simulink model "SF049A_LoaMgr"  (R2013b)
settings: Solver=FixedStepDiscrete  SolverMode=SingleTasking  StartTime=0.0  StopTime=1  FixedStep=0.002  RelTol=1e-3
values from neighbouring files (symbols this model uses):
  CURRMEASLOAMTGTNMASK_CNT_U08 = DataDict.Constant    [SF049A_LoaMgr_DataDict.m]
  IVTRLOAMTGTNMASK_CNT_U08 = DataDict.Constant    [SF049A_LoaMgr_DataDict.m]
  LOAMAXSLEW_ULSPERSEC_F32 = DataDict.Constant    [SF049A_LoaMgr_DataDict.m]
  LoaMgrCurrIvtrMtgtnRate = DataDict.Calibration    [SF049A_LoaMgr_DataDict.m]
  LoaMgrCurrIvtrMtgtnSca = DataDict.Calibration    [SF049A_LoaMgr_DataDict.m]
  LoaMgrCurrIvtrMtgtnScaZeroEna = DataDict.Calibration    [SF049A_LoaMgr_DataDict.m]
  LoaMgrCurrMeasIdptSig0Resp = DataDict.Calibration    [SF049A_LoaMgr_DataDict.m]
  LoaMgrCurrMeasIdptSig1Resp = DataDict.Calibration    [SF049A_LoaMgr_DataDict.m]
  LoaMgrCurrMeasIdptSig2Resp = DataDict.Calibration    [SF049A_LoaMgr_DataDict.m]
  LoaMgrCurrMeasIdptSigFltThd = DataDict.Calibration    [SF049A_LoaMgr_DataDict.m]
  LoaMgrCurrMeasMtgtnRate = DataDict.Calibration    [SF049A_LoaMgr_DataDict.m]
  LoaMgrCurrMeasMtgtnSca = DataDict.Calibration    [SF049A_LoaMgr_DataDict.m]
  LoaMgrCurrMeasMtgtnScaZeroEna = DataDict.Calibration    [SF049A_LoaMgr_DataDict.m]
  LoaMgrFadeOutStRate = DataDict.Calibration    [SF049A_LoaMgr_DataDict.m]
  LoaMgrHwTqIdptSig0NoTqLoaResp = DataDict.Calibration    [SF049A_LoaMgr_DataDict.m]
  LoaMgrHwTqIdptSig1NoTqLoaResp = DataDict.Calibration    [SF049A_LoaMgr_DataDict.m]
  LoaMgrHwTqIdptSig2Resp = DataDict.Calibration    [SF049A_LoaMgr_DataDict.m]
  LoaMgrHwTqIdptSig4Resp = DataDict.Calibration    [SF049A_LoaMgr_DataDict.m]
  LoaMgrHwTqIdptSigFltThd = DataDict.Calibration    [SF049A_LoaMgr_DataDict.m]
  LoaMgrHwTqLoaAvlResp = DataDict.Calibration    [SF049A_LoaMgr_DataDict.m]
  LoaMgrIvtrIdptSig0Resp = DataDict.Calibration    [SF049A_LoaMgr_DataDict.m]
  LoaMgrIvtrIdptSig1Resp = DataDict.Calibration    [SF049A_LoaMgr_DataDict.m]
  LoaMgrIvtrIdptSig2Resp = DataDict.Calibration    [SF049A_LoaMgr_DataDict.m]
  LoaMgrIvtrIdptSigFltThd = DataDict.Calibration    [SF049A_LoaMgr_DataDict.m]
  LoaMgrIvtrMtgtnRate = DataDict.Calibration    [SF049A_LoaMgr_DataDict.m]
  LoaMgrIvtrMtgtnSca = DataDict.Calibration    [SF049A_LoaMgr_DataDict.m]
  LoaMgrIvtrMtgtnScaZeroEna = DataDict.Calibration    [SF049A_LoaMgr_DataDict.m]
  LoaMgrLimdStRate = DataDict.Calibration    [SF049A_LoaMgr_DataDict.m]
  LoaMgrLimdStSca = DataDict.Calibration    [SF049A_LoaMgr_DataDict.m]
  LoaMgrMotAgAvlSnsrlsResp = DataDict.Calibration    [SF049A_LoaMgr_DataDict.m]
  LoaMgrMotAgIdptSig0NoSnsrlsResp = DataDict.Calibration    [SF049A_LoaMgr_DataDict.m]
  LoaMgrMotAgIdptSig1NoSnsrlsResp = DataDict.Calibration    [SF049A_LoaMgr_DataDict.m]
  LoaMgrMotAgIdptSig2Resp = DataDict.Calibration    [SF049A_LoaMgr_DataDict.m]
  LoaMgrMotAgIdptSig3Resp = DataDict.Calibration    [SF049A_LoaMgr_DataDict.m]
  LoaMgrMotAgIdptSigFltThd = DataDict.Calibration    [SF049A_LoaMgr_DataDict.m]
  LoaMgrMotAgMtgtnRate = DataDict.Calibration    [SF049A_LoaMgr_DataDict.m]
  LoaMgrMotAgMtgtnSca = DataDict.Calibration    [SF049A_LoaMgr_DataDict.m]
  LoaMgrMotAgMtgtnScaZeroEna = DataDict.Calibration    [SF049A_LoaMgr_DataDict.m]
  LOASCAONE_ULS_F32 = DataDict.Constant    [SF049A_LoaMgr_DataDict.m]
  LOASCAZERO_ULS_F32 = DataDict.Constant    [SF049A_LoaMgr_DataDict.m]
  LOASTIMDTSHTDWN_CNT_U08 = DataDict.Constant    [SF049A_LoaMgr_DataDict.m]
  LOASTNORM_CNT_U08 = DataDict.Constant    [SF049A_LoaMgr_DataDict.m]
  LOASTSWMTGTN_CNT_U08 = DataDict.Constant    [SF049A_LoaMgr_DataDict.m]
  MAXCURRMEASIDPTSIGALLWD_CNT_U08 = DataDict.Constant    [SF049A_LoaMgr_DataDict.m]
  MAXHWTQIDPTSIGALLWD_CNT_U08 = DataDict.Constant    [SF049A_LoaMgr_DataDict.m]
  MAXIVTRIDPTSIGALLWD_CNT_U08 = DataDict.Constant    [SF049A_LoaMgr_DataDict.m]
  MAXMOTAGMECLIDPTSIGALLWD_CNT_U08 = DataDict.Constant    [SF049A_LoaMgr_DataDict.m]
  NODEBSTEP_CNT_U16 = DataDict.Constant    [SF049A_LoaMgr_DataDict.m]
undefined symbols (not defined in the file or in its folder): LoaSt1, NtcNr1, NtcSts1, SigQlfr1
libraries: simulink x43, NxtrMin x4, NxtrMax x4, NxtrLim x2
(part 1 of 8)
settings Model: Creator=TZ5743  LastModifiedBy=dzvc93
settings SolverCC: AutoInsertRateTranBlk=on  InsertRTBMode=Always
settings DataIOCC: LimitDataPoints=off  SaveFormat=Structure  ReturnWorkspaceOutputs=on
settings OptimizationCC: BlockReduction=off  InlineParams=on  ZeroExternalMemoryAtStartup=off  ZeroInternalMemoryAtStartup=off  OptimizeModelRefInitCode=on  LifeSpan=1
settings DebuggingCC: SignalInfNanChecking=error  SignalRangeChecking=warning  UnderspecifiedInitializationDetection=Simplified  SolverPrmCheckMsg=error  InheritedTsInSrcMsg=error  DiscreteInheritContinuousMsg=error  SingleTaskRateTransMsg=error  TasksWithSamePriorityMsg=error  SigSpecEnsureSampleTimeMsg=error  CheckMatrixSingularityMsg=error  ParameterUnderflowMsg=error  ParameterPrecisionLossMsg=error  ParameterTunabilityLossMsg=error  FixptConstUnderflowMsg=warning  FixptConstOverflowMsg=warning  VectorMatrixConversionMsg=error  SignalLabelMismatchMsg=error  UnconnectedInputMsg=error  UnconnectedOutputMsg=error  UnconnectedLineMsg=error  SFcnCompatibilityMsg=error  UniqueDataStoreMsg=warning  BusObjectLabelMismatch=error  RootOutportRequireBusObject=error  AssertControl=DisableAll  ModelReferenceIOMsg=error  ModelReferenceVersionMismatchMessage=warning  ModelReferenceIOMismatchMessage=error  ModelReferenceCSMismatchMessage=warning  ModelReferenceDataLoggingMessage=error  StateNameClashWarn=warning  StrictBusMsg=ErrorOnBusTreatedAsVector  NonBusSignalsTreatedAsBus=error  SFUnexpectedBacktrackingDiag=error  SFInvalidInputDataAccessInChartInitDiag=error  SFNoUnconditionalDefaultTransitionDiag=error  SFTransitionOutsideNaturalParentDiag=error  SFUnconditionalTransitionShadowingDiag=error  SFUndirectedBroadcastEventsDiag=error
settings ModelReferenceCC: ModelReferenceNumInstancesAllowed=Single
settings RTWCC: SystemTargetFile=autosar.tlc  GenCodeOnly=on  TemplateMakefile=ert_default_tmf  Description=AUTOSAR  GenerateReport=on  ProcessScript=autosar_make_rtw_hook  LaunchReport=on
settings CodeAppCC: GenerateComments=off  IgnoreCustomStorageClasses=off  CustomSymbolStrType=$N$R$M  CustomSymbolStrBlkIO=$N$M  SimulinkBlockComments=off
settings STFCustomTargetCC: ParMdlRefBuildCompliant=on  CompOptLevelCompliant=on  IncludeMdlTerminateFcn=off  CombineOutputUpdateFcns=on  SuppressErrorStatus=on  ERTFirstTimeCompliant=on  ERTCustomFileBanners=on  SupportNonFinite=off  SupportComplex=off  SupportContinuousTime=off  SupportNonInlinedSFcns=off  MATLABClassNameForMDSCustomization=Simulink.SoftwareTarget.ERTCustomization  AutosarCompliant=on  GRTInterface=off  SystemTargetFile=autosar.tlc
settings ERTTargetCC: CodeReplacementLibrary=ANSI_C  ConcurrentExecutionCompliant=off  IncludeMdlTerminateFcn=off  SuppressErrorStatus=on  SupportNonFinite=off  SupportComplex=off  ModelStepFunctionPrototypeControlCompliant=off  CPPClassGenCompliant=off  AutosarCompliant=on  InlinedParameterPlacement=NonHierarchical  ERTCustomFileTemplate=example_file_process.tlc  EnableUserReplacementTypes=on

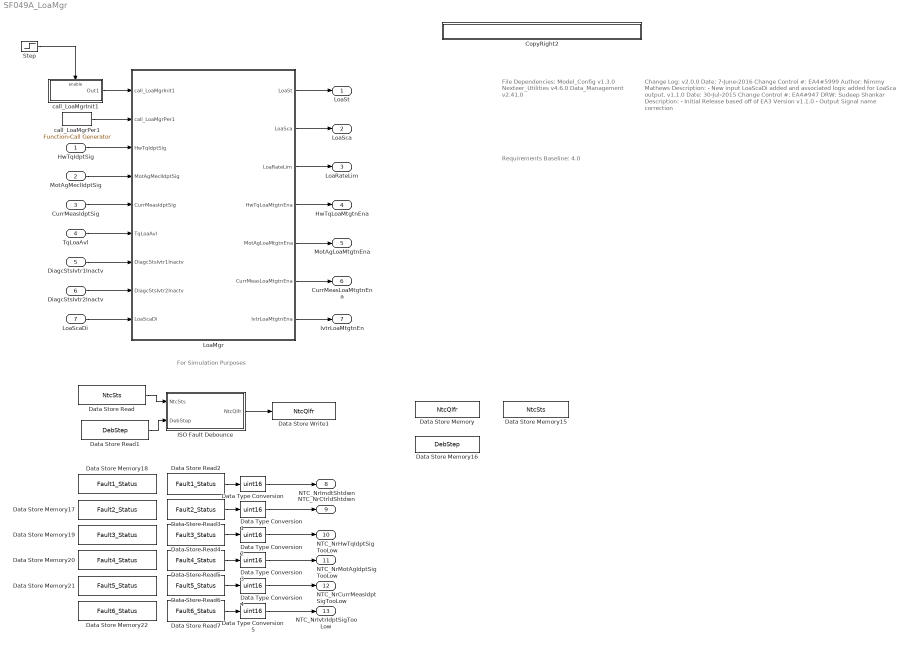
== system SF049A_LoaMgr ==
  note: File Dependencies:
      |
      | Model_Config v1.3.0
      | Nexteer_Utilities v4.6.0
      | Data_Management v2.41.0
  note: Requirements Baseline: 4.0
  note: Change Log:
      | v2.0.0
      | Date: 7-June-2016
      | Change Control #: 	EA4#5999
      | Author:  Nimmy Mathews
      | Description:
      | - New input LoaScaDi added and associated logic added for
      | LoaSca output.
      |
      | v1.1.0
      | Date: 30-Jul-2015
      | Change Control #: EA4#947
      | DRW:  Sudeep Shankar
      | Description:
      | - Initial Release based off of EA3 Version v1.1.0
      | - Output Signal name correction
  note: For Simulation Purposes
  HwTqIdptSig : Inport  RequirementInfo="{'linktype_rmi_doors' '0000bab3 (/E-STEER Core/SubSystem Specifications/Application Functions/SF049A Loss of Assist Manager)' '#SF049A_12' 'true' 'REQ:  SF049A_12' '' } %GIDa_c0ada7cc_2a84_41fc_944b_6b17ef65ea9c"
  MotAgMeclIdptSig : Inport  RequirementInfo="{'linktype_rmi_doors' '0000bab3 (/E-STEER Core/SubSystem Specifications/Application Functions/SF049A Loss of Assist Manager)' '#SF049A_14' 'true' 'REQ:  SF049A_14' '' } %GIDa_73372f4d_c568_47db_aad1_8b4638be1747"  Port=2
  CurrMeasIdptSig : Inport  RequirementInfo="{'linktype_rmi_doors' '0000bab3 (/E-STEER Core/SubSystem Specifications/Application Functions/SF049A Loss of Assist Manager)' '#SF049A_43' 'true' 'REQ:  SF049A_43' '' } %GIDa_84af9224_d287_43ff_b284_7e5ed6dfb324"  Port=3
  TqLoaAvl : Inport  RequirementInfo="{'linktype_rmi_doors' '0000bab3 (/E-STEER Core/SubSystem Specifications/Application Functions/SF049A Loss of Assist Manager)' '#SF049A_13' 'true' 'REQ:  SF049A_13' '' } %GIDa_93076217_93fd_4cef_a21d_6480a5a63a27"  Port=4
  DiagcStsIvtr1Inactv : Inport  RequirementInfo="{'linktype_rmi_doors' '0000bab3 (/E-STEER Core/SubSystem Specifications/Application Functions/SF049A Loss of Assist Manager)' '#SF049A_44' 'true' 'REQ:  SF049A_44' '' } %GIDa_3739eb85_24f0_476e_b882_4900d0ef3f73"  Port=5
  DiagcStsIvtr2Inactv : Inport  RequirementInfo="{'linktype_rmi_doors' '0000bab3 (/E-STEER Core/SubSystem Specifications/Application Functions/SF049A Loss of Assist Manager)' '#SF049A_184' 'true' 'REQ:  SF049A_184' '' } %GIDa_5f578b66_4982_413b_90dc_34bab3afd1d1"  Port=6
  LoaScaDi : Inport  RequirementInfo="{'linktype_rmi_doors' '0000bab3 (/E-STEER Core/SubSystem Specifications/Application Functions/SF049A Loss of Assist Manager)' '#SF049A_202' 'true' 'REQ:  SF049A_202' '' } %GIDa_13ee9f09_c993_4f8a_825d_b1ce3d1d2719"  Port=7
  CopyRight2 : Subsystem  Description=|  mask(Copyright Information){none=on}
      | Copyright info block.                                               
      |                                                                     
      | Place copyright information at the top of every subsystem in design.
      mask prompts: none "No parameters"
      mask help: Place copyright information at the top of every subsystem in design.
      mask Display:
      | NxtrConf = 'Nexteer Confidential';
      | 
      | sys = bdroot; %handle for the current model ("system")
      | first = get_param(sys,'Created');
      | if(isempty(first))
      |     first = datestr(now,'yyyy');
      | else
      |     first = first(end-3:end);  %year is last four digits
      | end
      | 
      | last = get_param(sys,'LastModifiedDate');
      | if isempty(last)
      |     last = datestr(now,'yyyy');
      | else
      |     last = last(end-3:end);
      | end
      | 
      | if strcmp(first,last)
      |     fprintf('%s -- Copyright %s Nexteer',NxtrConf,first)
      | else
      |     fprintf('%s -- %s%s- %s Nexteer',NxtrConf,char(169),first,last)
      | end
  Data Store Memory : DataStoreMemory  DataStoreName=NtcQlfr  OutDataTypeStr=uint8
  Data Store Memory15 : DataStoreMemory  DataStoreName=NtcSts  InitialValue=NtcSts1.NTCSTS_PREPASSD
  Data Store Memory16 : DataStoreMemory  DataStoreName=DebStep
  Data Store Memory17 : DataStoreMemory  DataStoreName=Fault2_Status  InitialValue=NtcSts1.NTCSTS_PASSD  OutDataTypeStr=Enum: NtcSts1
  Data Store Memory18 : DataStoreMemory  DataStoreName=Fault1_Status  InitialValue=NtcSts1.NTCSTS_PASSD  OutDataTypeStr=Enum: NtcSts1
  Data Store Memory19 : DataStoreMemory  DataStoreName=Fault3_Status  InitialValue=NtcSts1.NTCSTS_PASSD  OutDataTypeStr=Enum: NtcSts1
  Data Store Memory20 : DataStoreMemory  DataStoreName=Fault4_Status  InitialValue=NtcSts1.NTCSTS_PASSD  OutDataTypeStr=Enum: NtcSts1
  Data Store Memory21 : DataStoreMemory  DataStoreName=Fault5_Status  InitialValue=NtcSts1.NTCSTS_PASSD  OutDataTypeStr=Enum: NtcSts1
  Data Store Memory22 : DataStoreMemory  DataStoreName=Fault6_Status  InitialValue=NtcSts1.NTCSTS_PASSD  OutDataTypeStr=Enum: NtcSts1
  Data Store Read : DataStoreRead  DataStoreName=NtcSts  SampleTime=0.004
  Data Store Read1 : DataStoreRead  DataStoreName=DebStep  SampleTime=0.004
  Data Store Read2 : DataStoreRead  DataStoreName=Fault1_Status  SampleTime=.004
  Data Store Read3 : DataStoreRead  DataStoreName=Fault2_Status  SampleTime=.004
  Data Store Read4 : DataStoreRead  DataStoreName=Fault3_Status  SampleTime=.004
  Data Store Read5 : DataStoreRead  DataStoreName=Fault4_Status  SampleTime=.004
  Data Store Read6 : DataStoreRead  DataStoreName=Fault5_Status  SampleTime=.004
  Data Store Read7 : DataStoreRead  DataStoreName=Fault6_Status  SampleTime=0.004
  Data Store Write1 : DataStoreWrite  DataStoreName=NtcQlfr
  Data Type Conversion{,1..5} (6 alike) : DataTypeConversion  OutDataTypeStr=uint16
  ISO Fault Debounce : Subsystem
  LoaMgr : Subsystem
  Step : Step  Time=.001  Before=1  After=0  SampleTime=0
  call_LoaMgrInit1 : Subsystem  TreatAsAtomicUnit=on
  call_LoaMgrPer1 : simulink/Ports & Subsystems/Function-Call Generator  RequirementInfo="{'linktype_rmi_doors' '0000bab3 (/E-STEER Core/SubSystem Specifications/Application Functions/SF049A Loss of Assist Manager)' '#SF049A_28' 'true' 'REQ:  SF049A_28' '' } %GIDa_b45244a2_9238_4316_a679_a7195a05364e"  sample_time=0.004  numberOfIterations=1
  LoaSt : Outport  RequirementInfo="{'linktype_rmi_doors' '0000bab3 (/E-STEER Core/SubSystem Specifications/Application Functions/SF049A Loss of Assist Manager)' '#SF049A_16' 'true' 'REQ:  SF049A_16' '' } %GIDa_93bae52a_8cb1_4bd9_a2c4_d588b7d059cf"
  LoaSca : Outport  RequirementInfo="{'linktype_rmi_doors' '0000bab3 (/E-STEER Core/SubSystem Specifications/Application Functions/SF049A Loss of Assist Manager)' '#SF049A_17' 'true' 'REQ:  SF049A_17' '' } %GIDa_8c460775_12f6_4528_9f51_57ca189e85fc"  Port=2
  LoaRateLim : Outport  RequirementInfo="{'linktype_rmi_doors' '0000bab3 (/E-STEER Core/SubSystem Specifications/Application Functions/SF049A Loss of Assist Manager)' '#SF049A_18' 'true' 'REQ:  SF049A_18' '' } %GIDa_ffab9872_1ea4_4ffd_9e16_324c719cb008"  Port=3
  HwTqLoaMtgtnEna : Outport  RequirementInfo="{'linktype_rmi_doors' '0000bab3 (/E-STEER Core/SubSystem Specifications/Application Functions/SF049A Loss of Assist Manager)' '#SF049A_46' 'true' 'REQ:  SF049A_46' '' } %GIDa_b272817b_3ff3_4259_b745_ea4cd35b806a"  Port=4
  MotAgLoaMtgtnEna : Outport  RequirementInfo="{'linktype_rmi_doors' '0000bab3 (/E-STEER Core/SubSystem Specifications/Application Functions/SF049A Loss of Assist Manager)' '#SF049A_47' 'true' 'REQ:  SF049A_47' '' } %GIDa_98224876_72c1_4d11_a238_725dcb00f091"  Port=5
  CurrMeasLoaMtgtnEna : Outport  RequirementInfo="{'linktype_rmi_doors' '0000bab3 (/E-STEER Core/SubSystem Specifications/Application Functions/SF049A Loss of Assist Manager)' '#SF049A_48' 'true' 'REQ:  SF049A_48' '' } %GIDa_771c3727_c0e3_4c42_9260_a180eb374e5c"  Port=6
  IvtrLoaMtgtnEn : Outport  RequirementInfo="{'linktype_rmi_doors' '0000bab3 (/E-STEER Core/SubSystem Specifications/Application Functions/SF049A Loss of Assist Manager)' '#SF049A_49' 'true' 'REQ:  SF049A_49' '' } %GIDa_ccb9de9c_ade8_4e48_bfad_57a91e3cbf19"  Port=7
  NTC_NrImdtShtdwn : Outport  Port=8
  NTC_NrCtrldShtdwn : Outport  Port=9
  NTC_NrHwTqIdptSigTooLow : Outport  Port=10
  NTC_NrMotAgIdptSigTooLow : Outport  Port=11
  NTC_NrCurrMeasIdptSigTooLow : Outport  Port=12
  NTC_NrIvtrIdptSigTooLow : Outport  Port=13
  wires:
  HwTqIdptSig/1 -> LoaMgr/3(HwTqIdptSig)
  MotAgMeclIdptSig/1 -> LoaMgr/4(MotAgMeclIdptSig)
  CurrMeasIdptSig/1 -> LoaMgr/5(CurrMeasIdptSig)
  DiagcStsIvtr1Inactv/1 -> LoaMgr/7(DiagcStsIvtr1Inactv)
  TqLoaAvl/1 -> LoaMgr/6(TqLoaAvl)
  DiagcStsIvtr2Inactv/1 -> LoaMgr/8(DiagcStsIvtr2Inactv)
  LoaMgr/7(IvtrLoaMtgtnEna) -> IvtrLoaMtgtnEn/1
  LoaMgr/6(CurrMeasLoaMtgtnEna) -> CurrMeasLoaMtgtnEna/1
  LoaMgr/5(MotAgLoaMtgtnEna) -> MotAgLoaMtgtnEna/1
  LoaMgr/4(HwTqLoaMtgtnEna) -> HwTqLoaMtgtnEna/1
  LoaMgr/3(LoaRateLim) -> LoaRateLim/1
  LoaMgr/2(LoaSca) -> LoaSca/1
  LoaMgr/1(LoaSt) -> LoaSt/1
  call_LoaMgrPer1/1 -> LoaMgr/2(call_LoaMgrPer1)
  call_LoaMgrInit1/1(Out1) -> LoaMgr/1(call_LoaMgrInit1)
  Step/1 -> call_LoaMgrInit1/Enable
  Data Store Read2/1 -> Data Type Conversion/1
  Data Type Conversion/1 -> NTC_NrImdtShtdwn/1
  Data Store Read3/1 -> Data Type Conversion1/1
  Data Type Conversion1/1 -> NTC_NrCtrldShtdwn/1
  Data Store Read4/1 -> Data Type Conversion2/1
  Data Type Conversion2/1 -> NTC_NrHwTqIdptSigTooLow/1
  Data Type Conversion3/1 -> NTC_NrMotAgIdptSigTooLow/1
  Data Type Conversion4/1 -> NTC_NrCurrMeasIdptSigTooLow/1
  Data Store Read5/1 -> Data Type Conversion3/1
  Data Store Read6/1 -> Data Type Conversion4/1
  Data Type Conversion5/1 -> NTC_NrIvtrIdptSigTooLow/1
  Data Store Read7/1 -> Data Type Conversion5/1
  ISO Fault Debounce/1(NtcQlfr) -> Data Store Write1/1
  Data Store Read/1 -> ISO Fault Debounce/1(NtcSts)
  Data Store Read1/1 -> ISO Fault Debounce/2(DebStep)
  LoaScaDi/1 -> LoaMgr/9(LoaScaDi)

== system SF049A_LoaMgr/CopyRight2 ==

== system SF049A_LoaMgr/ISO Fault Debounce ==
  note: Note:
      |
      | - "ISO Fault Debounce Design" Simulink block intent to use here for Simulation purpose only. Do not Code this block
  NtcSts : Inport
  DebStep : Inport  Port=2
  Constant : Constant  Value=false
  CopyRight2 : Subsystem  Description=|  mask(Copyright Information){none=on}
      | Copyright info block.                                               
      |                                                                     
      | Place copyright information at the top of every subsystem in design.
      mask prompts: none "No parameters"
      mask help: Place copyright information at the top of every subsystem in design.
      mask Display:
      | NxtrConf = 'Nexteer Confidential';
      | 
      | sys = bdroot; %handle for the current model ("system")
      | first = get_param(sys,'Created');
      | first = first(end-3:end);  %year is last four digits
      | 
      | last = get_param(sys,'LastModifiedDate');
      | if isempty(last)
      |     last = datestr(now,'yyyy');
      | else
      |     last = last(end-3:end);
      | end
      | 
      | if strcmp(first,last)
      |     fprintf('%s -- Copyright %s Nexteer',NxtrConf,first)
      | else
      |     fprintf('%s -- %s%s- %s Nexteer',NxtrConf,char(169),first,last)
      | end
  Data Type Conversion : DataTypeConversion
  DiagMgr : Subsystem  RequirementInfo="{'linktype_rmi_doors' '00007fee (/E-STEER Core/SubSystem Specifications/Application Functions/SF004B Assist Summation and Limiting- Current)' '#SF004B_271' 'true' 'REQ:  SF004B_271' '' ; 'linktype_rmi_doors' '00007fee (/E-STEER Core/SubSystem Specifications/Application Functions/SF004B Assist Summation and Limiting- Current)' '#SF004B_270' 'true' 'REQ:  SF004B_270' '' ; 'linktype_rmi_doors' '00007fee (/E-STEER Core/SubSystem Specifications/Application Functions/SF004B Assist Summation and Limiting- Current)' '#SF004B_272' 'true' 'REQ:  SF004B_272' '' ; 'linktype_rmi_doors' '00007fee (/E-STEER Core/SubSystem Specifications/Application Functions/SF004B Assist Summation and Limiting- Current)' '#SF004B_273' 'true' 'REQ:  SF004B_273' '' } %GIDa_8ac3e521_cc41_436f_a252_177cc8f755d2"
  Ground : Ground
  Scope2 : Scope
      settings: SaveName=ScopeData2
  Terminator : Terminator
  NtcQlfr : Outport
  wires:
  Ground/1 -> DiagMgr/3(SvcClr)
  DebStep/1 -> DiagMgr/2(DebStep), Scope2/1
  NtcSts/1 -> DiagMgr/1(NtcSts)
  Constant/1 -> DiagMgr/4(Recoverable)
  Data Type Conversion/1 -> NtcQlfr/1
  DiagMgr/1(Qualifier) -> Data Type Conversion/1
  DiagMgr/2(ErrAcc) -> Terminator/1

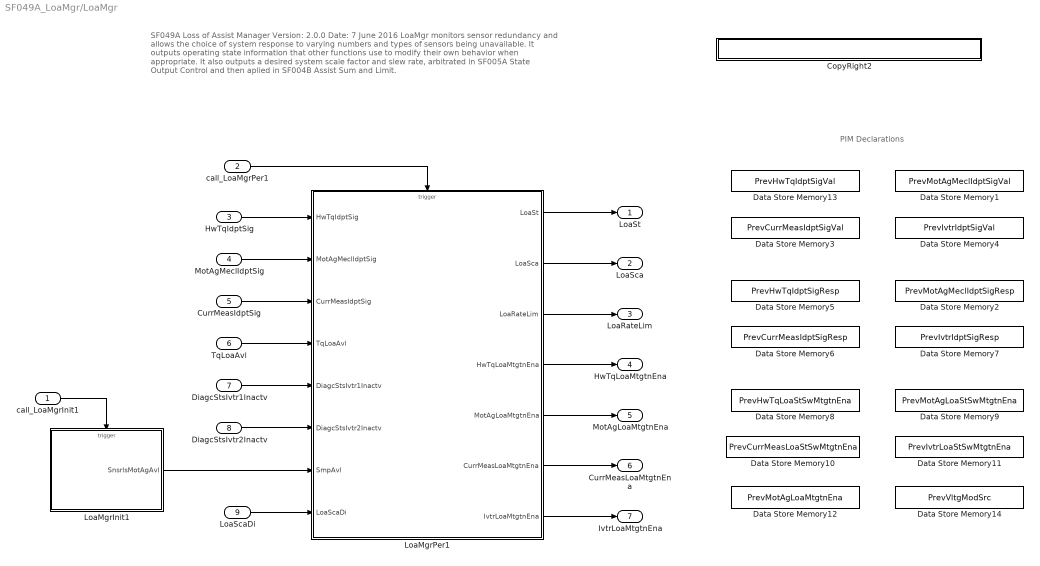
== system SF049A_LoaMgr/LoaMgr ==
  note: PIM Declarations
  note: SF049A  Loss of Assist Manager       Version: 2.0.0                                                       Date:  7 June 2016
      |
      | LoaMgr monitors sensor redundancy and allows the choice of system response to varying numbers and types of sensors being unavailable.  It
      | outputs operating state information that other functions use to modify their own behavior when appropriate.  It also outputs a desired system
      | scale factor and slew rate, arbitrated in SF005A State Output Control and then aplied in SF004B Assist Sum and Limit.
  call_LoaMgrInit1 : Inport
  call_LoaMgrPer1 : Inport  Port=2
  HwTqIdptSig : Inport  RequirementInfo="{'linktype_rmi_doors' '0000bab3 (/E-STEER Core/SubSystem Specifications/Application Functions/SF049A Loss of Assist Manager)' '#SF049A_12' 'true' 'REQ:  SF049A_12' '' } %GIDa_738d9608_1f11_48d9_b5fb_db6b875da4f0"  Port=3
  MotAgMeclIdptSig : Inport  RequirementInfo="{'linktype_rmi_doors' '0000bab3 (/E-STEER Core/SubSystem Specifications/Application Functions/SF049A Loss of Assist Manager)' '#SF049A_14' 'true' 'REQ:  SF049A_14' '' } %GIDa_2a624495_d7cc_4d20_92e8_f9f8d9f5c9c4"  Port=4
  CurrMeasIdptSig : Inport  RequirementInfo="{'linktype_rmi_doors' '0000bab3 (/E-STEER Core/SubSystem Specifications/Application Functions/SF049A Loss of Assist Manager)' '#SF049A_43' 'true' 'REQ:  SF049A_43' '' } %GIDa_91d29884_2257_4923_b9cb_724eaa988704"  Port=5
  TqLoaAvl : Inport  RequirementInfo="{'linktype_rmi_doors' '0000bab3 (/E-STEER Core/SubSystem Specifications/Application Functions/SF049A Loss of Assist Manager)' '#SF049A_13' 'true' 'REQ:  SF049A_13' '' } %GIDa_67da4e6f_783e_4b7f_b2da_bafe95c201fd"  Port=6
  DiagcStsIvtr1Inactv : Inport  RequirementInfo="{'linktype_rmi_doors' '0000bab3 (/E-STEER Core/SubSystem Specifications/Application Functions/SF049A Loss of Assist Manager)' '#SF049A_44' 'true' 'REQ:  SF049A_44' '' } %GIDa_d2a02f01_0f9a_4a35_b83d_8146e48af58f"  Port=7
  DiagcStsIvtr2Inactv : Inport  RequirementInfo="{'linktype_rmi_doors' '0000bab3 (/E-STEER Core/SubSystem Specifications/Application Functions/SF049A Loss of Assist Manager)' '#SF049A_184' 'true' 'REQ:  SF049A_184' '' } %GIDa_6476a35b_29d3_4546_be5a_73a3a90db49d"  Port=8
  LoaScaDi : Inport  RequirementInfo="{'linktype_rmi_doors' '0000bab3 (/E-STEER Core/SubSystem Specifications/Application Functions/SF049A Loss of Assist Manager)' '#SF049A_202' 'true' 'REQ:  SF049A_202' '' } %GIDa_837ddbd3_ccbc_45e5_bb35_092182484950"  Port=9
  CopyRight2 : Subsystem  Description=|  mask(Copyright Information){none=on}
      | Copyright info block.                                               
      |                                                                     
      | Place copyright information at the top of every subsystem in design.
      mask prompts: none "No parameters"
      mask help: Place copyright information at the top of every subsystem in design.
      mask Display:
      | NxtrConf = 'Nexteer Confidential';
      | 
      | sys = bdroot; %handle for the current model ("system")
      | first = get_param(sys,'Created');
      | first = first(end-3:end);  %year is last four digits
      | 
      | last = get_param(sys,'LastModifiedDate');
      | if isempty(last)
      |     last = datestr(now,'yyyy');
      | else
      |     last = last(end-3:end);
      | end
      | 
      | if strcmp(first,last)
      |     fprintf('%s -- Copyright %s Nexteer',NxtrConf,first)
      | else
      |     fprintf('%s -- %s%s- %s Nexteer',NxtrConf,char(169),first,last)
      | end
  Data Store Memory1 : DataStoreMemory  DataStoreName=PrevMotAgMeclIdptSigVal  StateMustResolveToSignalObject=on
  Data Store Memory10 : DataStoreMemory  DataStoreName=PrevCurrMeasLoaStSwMtgtnEna  StateMustResolveToSignalObject=on
  Data Store Memory11 : DataStoreMemory  DataStoreName=PrevIvtrLoaStSwMtgtnEna  StateMustResolveToSignalObject=on
  Data Store Memory12 : DataStoreMemory  DataStoreName=PrevMotAgLoaMtgtnEna  StateMustResolveToSignalObject=on
  Data Store Memory13 : DataStoreMemory  DataStoreName=PrevHwTqIdptSigVal  StateMustResolveToSignalObject=on
  Data Store Memory14 : DataStoreMemory  DataStoreName=PrevVltgModSrc  StateMustResolveToSignalObject=on
  Data Store Memory2 : DataStoreMemory  DataStoreName=PrevMotAgMeclIdptSigResp  StateMustResolveToSignalObject=on
  Data Store Memory3 : DataStoreMemory  DataStoreName=PrevCurrMeasIdptSigVal  StateMustResolveToSignalObject=on
  Data Store Memory4 : DataStoreMemory  DataStoreName=PrevIvtrIdptSigVal  StateMustResolveToSignalObject=on
  Data Store Memory5 : DataStoreMemory  DataStoreName=PrevHwTqIdptSigResp  StateMustResolveToSignalObject=on
  Data Store Memory6 : DataStoreMemory  DataStoreName=PrevCurrMeasIdptSigResp  StateMustResolveToSignalObject=on
  Data Store Memory7 : DataStoreMemory  DataStoreName=PrevIvtrIdptSigResp  StateMustResolveToSignalObject=on
  Data Store Memory8 : DataStoreMemory  DataStoreName=PrevHwTqLoaStSwMtgtnEna  StateMustResolveToSignalObject=on
  Data Store Memory9 : DataStoreMemory  DataStoreName=PrevMotAgLoaStSwMtgtnEna  StateMustResolveToSignalObject=on
  LoaMgrInit1 : Subsystem  TreatAsAtomicUnit=on
  LoaMgrPer1 : Subsystem
  LoaSt : Outport  RequirementInfo="{'linktype_rmi_doors' '0000bab3 (/E-STEER Core/SubSystem Specifications/Application Functions/SF049A Loss of Assist Manager)' '#SF049A_16' 'true' 'REQ:  SF049A_16' '' } %GIDa_bd422f72_73e1_4e92_bf3c_ebd4d43c1ed1"
  LoaSca : Outport  RequirementInfo="{'linktype_rmi_doors' '0000bab3 (/E-STEER Core/SubSystem Specifications/Application Functions/SF049A Loss of Assist Manager)' '#SF049A_17' 'true' 'REQ:  SF049A_17' '' } %GIDa_0436fd41_dcd9_46ab_bfae_9f19b4d66e99"  Port=2
  LoaRateLim : Outport  RequirementInfo="{'linktype_rmi_doors' '0000bab3 (/E-STEER Core/SubSystem Specifications/Application Functions/SF049A Loss of Assist Manager)' '#SF049A_18' 'true' 'REQ:  SF049A_18' '' } %GIDa_faf9e70c_66ed_4dc9_a19c_b08600e4b753"  Port=3
  HwTqLoaMtgtnEna : Outport  RequirementInfo="{'linktype_rmi_doors' '0000bab3 (/E-STEER Core/SubSystem Specifications/Application Functions/SF049A Loss of Assist Manager)' '#SF049A_46' 'true' 'REQ:  SF049A_46' '' } %GIDa_7abc6027_7519_46d6_983d_70d6c7f8cf42"  Port=4
  MotAgLoaMtgtnEna : Outport  RequirementInfo="{'linktype_rmi_doors' '0000bab3 (/E-STEER Core/SubSystem Specifications/Application Functions/SF049A Loss of Assist Manager)' '#SF049A_47' 'true' 'REQ:  SF049A_47' '' } %GIDa_7e3009d4_7a2d_4dd4_8406_9bc55f402990"  Port=5
  CurrMeasLoaMtgtnEna : Outport  RequirementInfo="{'linktype_rmi_doors' '0000bab3 (/E-STEER Core/SubSystem Specifications/Application Functions/SF049A Loss of Assist Manager)' '#SF049A_48' 'true' 'REQ:  SF049A_48' '' } %GIDa_08006616_1462_4391_8737_64914ece57a0"  Port=6
  IvtrLoaMtgtnEna : Outport  RequirementInfo="{'linktype_rmi_doors' '0000bab3 (/E-STEER Core/SubSystem Specifications/Application Functions/SF049A Loss of Assist Manager)' '#SF049A_49' 'true' 'REQ:  SF049A_49' '' } %GIDa_5c05b292_5d23_4a61_89b4_07b4a41f7227"  Port=7
  wires:
  LoaMgrInit1/1(SnsrlsMotAgAvl) -> LoaMgrPer1/7(SmpAvl)
  call_LoaMgrInit1/1 -> LoaMgrInit1/Trigger
  DiagcStsIvtr2Inactv/1 -> LoaMgrPer1/6(DiagcStsIvtr2Inactv)
  CurrMeasIdptSig/1 -> LoaMgrPer1/3(CurrMeasIdptSig)
  DiagcStsIvtr1Inactv/1 -> LoaMgrPer1/5(DiagcStsIvtr1Inactv)
  TqLoaAvl/1 -> LoaMgrPer1/4(TqLoaAvl)
  HwTqIdptSig/1 -> LoaMgrPer1/1(HwTqIdptSig)
  MotAgMeclIdptSig/1 -> LoaMgrPer1/2(MotAgMeclIdptSig)
  call_LoaMgrPer1/1 -> LoaMgrPer1/Trigger
  LoaMgrPer1/7(IvtrLoaMtgtnEna) -> IvtrLoaMtgtnEna/1
  LoaMgrPer1/6(CurrMeasLoaMtgtnEna) -> CurrMeasLoaMtgtnEna/1
  LoaMgrPer1/5(MotAgLoaMtgtnEna) -> MotAgLoaMtgtnEna/1
  LoaMgrPer1/4(HwTqLoaMtgtnEna) -> HwTqLoaMtgtnEna/1
  LoaMgrPer1/3(LoaRateLim) -> LoaRateLim/1
  LoaMgrPer1/2(LoaSca) -> LoaSca/1
  LoaMgrPer1/1(LoaSt) -> LoaSt/1
  LoaScaDi/1 -> LoaMgrPer1/8(LoaScaDi)

== system SF049A_LoaMgr/call_LoaMgrInit1 ==
  Enable : EnablePort
  Function-Call Generator : simulink/Ports & Subsystems/Function-Call Generator  sample_time=.004  numberOfIterations=1
  Out1 : Outport
  wires:
  Function-Call Generator/1 -> Out1/1

== system SF049A_LoaMgr/ISO Fault Debounce/CopyRight2 ==

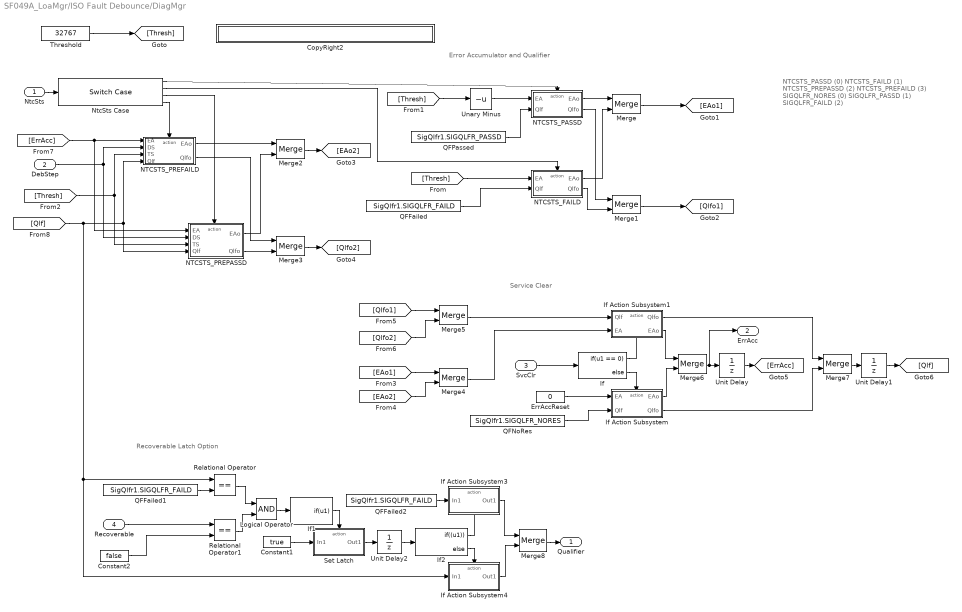
== system SF049A_LoaMgr/ISO Fault Debounce/DiagMgr ==
  note: NTCSTS_PASSD         (0)
      | NTCSTS_FAILD           (1)
      | NTCSTS_PREPASSD  (2)
      | NTCSTS_PREFAILD    (3)
      |
      | SIGQLFR_NORES       (0)
      | SIGQLFR_PASSD        (1)
      | SIGQLFR_FAILD          (2)
  note: Error Accumulator and Qualifier
  note: Service Clear
  note: Recoverable Latch Option
  NtcSts : Inport
  DebStep : Inport  Port=2
  SvcClr : Inport  Port=3
  Recoverable : Inport  Port=4
  Constant1 : Constant  Value=true  OutDataTypeStr=boolean
  Constant2 : Constant  Value=false  OutDataTypeStr=boolean
  CopyRight2 : Subsystem  Description=|  mask(Copyright Information){none=on}
      | Copyright info block.                                               
      |                                                                     
      | Place copyright information at the top of every subsystem in design.
      mask prompts: none "No parameters"
      mask help: Place copyright information at the top of every subsystem in design.
      mask Display:
      | NxtrConf = 'Nexteer Confidential';
      | 
      | sys = bdroot; %handle for the current model ("system")
      | first = get_param(sys,'Created');
      | first = first(end-3:end);  %year is last four digits
      | 
      | last = get_param(sys,'LastModifiedDate');
      | if isempty(last)
      |     last = datestr(now,'yyyy');
      | else
      |     last = last(end-3:end);
      | end
      | 
      | if strcmp(first,last)
      |     fprintf('%s -- Copyright %s Nexteer',NxtrConf,first)
      | else
      |     fprintf('%s -- %s%s- %s Nexteer',NxtrConf,char(169),first,last)
      | end
  ErrAccReset : Constant  Value=0
  If : If  IfExpression=u1 == 0
  If Action Subsystem : Subsystem  TreatAsAtomicUnit=on
  If Action Subsystem1 : Subsystem  TreatAsAtomicUnit=on
  If Action Subsystem3 : Subsystem  TreatAsAtomicUnit=on
  If Action Subsystem4 : Subsystem  TreatAsAtomicUnit=on
  If1 : If  IfExpression=u1  ShowElse=off
  If2 : If  IfExpression=(u1)
  Logical Operator : Logic  AllPortsSameDT=off  OutDataTypeStr=boolean
  Merge{,1..8} (9 alike) : Merge
  NTCSTS_FAILD : Subsystem  TreatAsAtomicUnit=on
  NTCSTS_PASSD : Subsystem  TreatAsAtomicUnit=on
  NTCSTS_PREFAILD : Subsystem  TreatAsAtomicUnit=on
  NTCSTS_PREPASSD : Subsystem  TreatAsAtomicUnit=on
  NtcSts Case : SwitchCase  CaseConditions={NtcSts1.NTCSTS_PASSD,NtcSts1.NTCSTS_FAILD,NtcSts1.NTCSTS_PREPASSD,NtcSts1.NTCSTS_PREFAILD}  ShowDefaultCase=off
  QFFailed : Constant  Value=SigQlfr1.SIGQLFR_FAILD  OutDataTypeStr=Enum: SigQlfr1
  QFFailed1 : Constant  Value=SigQlfr1.SIGQLFR_FAILD  OutDataTypeStr=Enum: SigQlfr1
  QFFailed2 : Constant  Value=SigQlfr1.SIGQLFR_FAILD  OutDataTypeStr=Enum: SigQlfr1
  QFNoRes : Constant  Value=SigQlfr1.SIGQLFR_NORES  OutDataTypeStr=Enum: SigQlfr1
  QFPassed : Constant  Value=SigQlfr1.SIGQLFR_PASSD  OutDataTypeStr=Enum: SigQlfr1
  Relational Operator : RelationalOperator  Operator===  OutDataTypeStr=boolean
      settings: AttributesFormatString=Qualifier Failed
  Relational Operator1 : RelationalOperator  Operator===  OutDataTypeStr=boolean
      settings: AttributesFormatString=Recoverable False
  Set Latch : Subsystem  TreatAsAtomicUnit=on
  Threshold : Constant  Value=32767
  Unary Minus : UnaryMinus
  Unit Delay : UnitDelay  SampleTime=-1
  Unit Delay1 : UnitDelay  InitialCondition=SigQlfr1.SIGQLFR_NORES  SampleTime=-1  StateName=SigQlfr1
  Unit Delay2 : UnitDelay  SampleTime=-1
  Qualifier : Outport
  ErrAcc : Outport  Port=2
  wires:
  DebStep/1 -> NTCSTS_PREPASSD/2(DS), NTCSTS_PREFAILD/2(DS)
  NtcSts Case/3 -> NTCSTS_PREPASSD/Action
  If/2 -> If Action Subsystem/Action
  QFPassed/1 -> NTCSTS_PASSD/2(Qlf)
  If2/1 -> If Action Subsystem3/Action
  If2/2 -> If Action Subsystem4/Action
  [Thresh] -> NTCSTS_FAILD/1(EA)
  QFFailed/1 -> NTCSTS_FAILD/2(Qlf)
  If Action Subsystem4/1(Out1) -> Merge8/2
  Merge8/1 -> Qualifier/1
  QFFailed2/1 -> If Action Subsystem3/1(In1)
  Unit Delay2/1 -> If2/1
  NtcSts Case/1 -> NTCSTS_PASSD/Action
  NtcSts Case/4 -> NTCSTS_PREFAILD/Action
  SvcClr/1 -> If/1
  NtcSts Case/2 -> NTCSTS_FAILD/Action
  [Thresh] -> Unary Minus/1
  [Thresh] -> NTCSTS_PREPASSD/3(TS), NTCSTS_PREFAILD/3(TS)
  NTCSTS_PREFAILD/2(Qlfo) -> Merge3/1
  [ErrAcc] -> NTCSTS_PREPASSD/1(EA), NTCSTS_PREFAILD/1(EA)
  NTCSTS_PREPASSD/1(EAo) -> Merge2/2
  NTCSTS_FAILD/1(EAo) -> Merge/2
  NTCSTS_FAILD/2(Qlfo) -> Merge1/2
  If Action Subsystem3/1(Out1) -> Merge8/1
  [Qlfo1] -> Merge5/1
  NTCSTS_PREPASSD/2(Qlfo) -> Merge3/2
  NTCSTS_PREFAILD/1(EAo) -> Merge2/1
  [Qlfo2] -> Merge5/2
  [EAo1] -> Merge4/1
  [Qlf] -> Relational Operator/1, If Action Subsystem4/1(In1), NTCSTS_PREFAILD/4(Qlf), NTCSTS_PREPASSD/4(Qlf)
  [EAo2] -> Merge4/2
  Merge/1 -> [EAo1]
  ErrAccReset/1 -> If Action Subsystem/1(EA)
  QFNoRes/1 -> If Action Subsystem/2(Qlf)
  Merge6/1 -> ErrAcc/1, Unit Delay/1
  If Action Subsystem1/2(EAo) -> Merge6/1
  Merge4/1 -> If Action Subsystem1/2(EA)
  If/1 -> If Action Subsystem1/Action
  If Action Subsystem1/1(Qlfo) -> Merge7/1
  NTCSTS_PASSD/2(Qlfo) -> Merge1/1
  Threshold/1 -> [Thresh]
  If Action Subsystem/1(EAo) -> Merge6/2
  NTCSTS_PASSD/1(EAo) -> Merge/1
  If Action Subsystem/2(Qlfo) -> Merge7/2
  Merge1/1 -> [Qlfo1]
  Merge2/1 -> [EAo2]
  Merge3/1 -> [Qlfo2]
  Merge5/1 -> If Action Subsystem1/1(Qlf)
  NtcSts/1 -> NtcSts Case/1
  Unit Delay/1 -> [ErrAcc]
  Unit Delay1/1 -> [Qlf]
  Merge7/1 -> Unit Delay1/1
  Relational Operator/1 -> Logical Operator/1
  Relational Operator1/1 -> Logical Operator/2
  Constant2/1 -> Relational Operator1/2
  Logical Operator/1 -> If1/1
  If1/1 -> Set Latch/Action
  Constant1/1 -> Set Latch/1(In1)
  QFFailed1/1 -> Relational Operator/2
  Set Latch/1(Out1) -> Unit Delay2/1
  Recoverable/1 -> Relational Operator1/1
  Unary Minus/1 -> NTCSTS_PASSD/1(EA)

== system SF049A_LoaMgr/LoaMgr/CopyRight2 ==

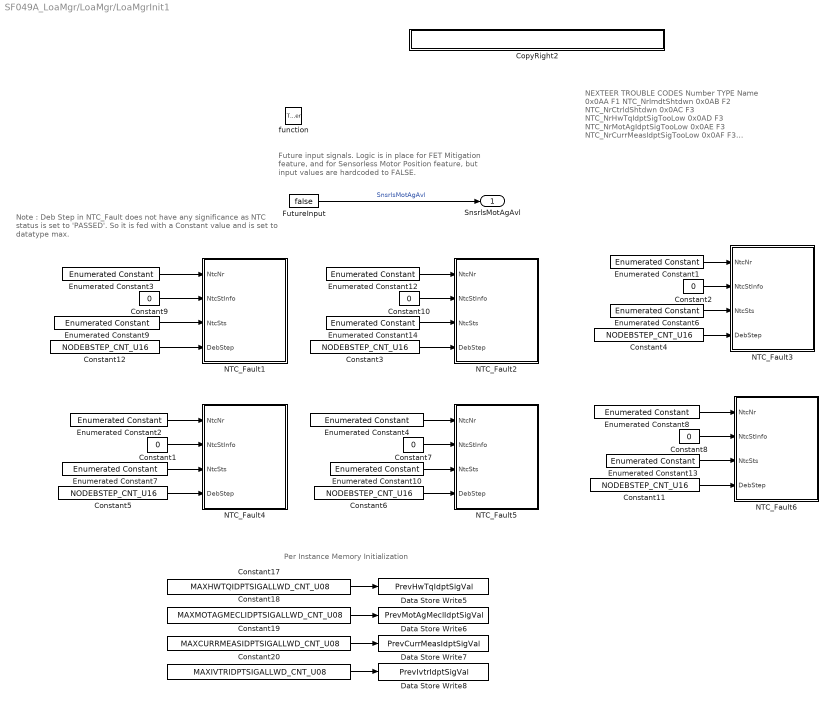
== system SF049A_LoaMgr/LoaMgr/LoaMgrInit1 ==
  note: Note : Deb Step in NTC_Fault does not have any significance as
      | NTC status is set to 'PASSED'. So it is fed with a Constant value and
      | is set to datatype max.
  note: Future input signals.  Logic is in place for FET Mitigation
      | feature, and for Sensorless Motor Position feature,
      | but input values are hardcoded to FALSE.
  note: NEXTEER TROUBLE CODES
      | Number  TYPE   Name
      |  0x0AA      F1      NTC_NrImdtShtdwn
      |  0x0AB      F2      NTC_NrCtrldShtdwn
      |  0x0AC      F3      NTC_NrHwTqIdptSigTooLow
      |  0x0AD      F3      NTC_NrMotAgIdptSigTooLow
      |  0x0AE      F3      NTC_NrCurrMeasIdptSigTooLow
      |  0x0AF      F3      NTC_NrIvtrIdptSigTooLow
  note: Per Instance Memory Initialization
  function : TriggerPort  TriggerType=function-call
  Constant{1..2,7..10} (6 alike) : Constant  Value=0
  Constant{3..6,11..12} (6 alike) : Constant  Value=NODEBSTEP_CNT_U16
  Constant17 : Constant  RequirementInfo={} %GIDa_802eeff3_527a_45d1_bc70_a03443e7aa2c  Value=MAXHWTQIDPTSIGALLWD_CNT_U08  OutDataTypeStr=uint8
  Constant18 : Constant  RequirementInfo={} %GIDa_be72a58d_a3b8_4979_8748_805cdbd241be  Value=MAXMOTAGMECLIDPTSIGALLWD_CNT_U08  OutDataTypeStr=uint8
  Constant19 : Constant  RequirementInfo={} %GIDa_a19eae2c_6945_424b_b4d9_f313d764a177  Value=MAXCURRMEASIDPTSIGALLWD_CNT_U08  OutDataTypeStr=uint8
  Constant20 : Constant  RequirementInfo={} %GIDa_98abaa99_050a_496b_a139_9c0215867b93  Value=MAXIVTRIDPTSIGALLWD_CNT_U08  OutDataTypeStr=uint8
  CopyRight2 : Subsystem  Description=|  mask(Copyright Information){none=on}
      | Copyright info block.                                               
      |                                                                     
      | Place copyright information at the top of every subsystem in design.
      mask prompts: none "No parameters"
      mask help: Place copyright information at the top of every subsystem in design.
      mask Display:
      | NxtrConf = 'Nexteer Confidential';
      | 
      | sys = bdroot; %handle for the current model ("system")
      | first = get_param(sys,'Created');
      | first = first(end-3:end);  %year is last four digits
      | 
      | last = get_param(sys,'LastModifiedDate');
      | if isempty(last)
      |     last = datestr(now,'yyyy');
      | else
      |     last = last(end-3:end);
      | end
      | 
      | if strcmp(first,last)
      |     fprintf('%s -- Copyright %s Nexteer',NxtrConf,first)
      | else
      |     fprintf('%s -- %s%s- %s Nexteer',NxtrConf,char(169),first,last)
      | end
  Data Store Write5 : DataStoreWrite  RequirementInfo={} %GIDa_bdfcf81e_29a0_4350_885d_bce6caf2931a  DataStoreName=PrevHwTqIdptSigVal
  Data Store Write6 : DataStoreWrite  RequirementInfo={} %GIDa_536911fe_ac58_4e6a_8b36_db2e3d7c797d  DataStoreName=PrevMotAgMeclIdptSigVal
  Data Store Write7 : DataStoreWrite  RequirementInfo={} %GIDa_e67b9b72_1ee7_4273_a0a3_24fc29f0a974  DataStoreName=PrevCurrMeasIdptSigVal
  Data Store Write8 : DataStoreWrite  RequirementInfo={} %GIDa_ffbd528d_1eac_43cd_ae27_aa0faef492c4  DataStoreName=PrevIvtrIdptSigVal
  Enumerated Constant1 : simulink/Sources/Enumerated Constant  OutDataTypeStr=Enum: NtcNr1  Value=NtcNr1.NTCNR_0X0AC  SampleTime=inf
  Enumerated Constant12 : simulink/Sources/Enumerated Constant  OutDataTypeStr=Enum: NtcNr1  Value=NtcNr1.NTCNR_0X0AB  SampleTime=inf
  Enumerated Constant2 : simulink/Sources/Enumerated Constant  OutDataTypeStr=Enum: NtcNr1  Value=NtcNr1.NTCNR_0X0AD  SampleTime=inf
  Enumerated Constant3 : simulink/Sources/Enumerated Constant  OutDataTypeStr=Enum: NtcNr1  Value=NtcNr1.NTCNR_0X0AA  SampleTime=inf
  Enumerated Constant4 : simulink/Sources/Enumerated Constant  OutDataTypeStr=Enum: NtcNr1  Value=NtcNr1.NTCNR_0X0AE  SampleTime=inf
  Enumerated Constant8 : simulink/Sources/Enumerated Constant  OutDataTypeStr=Enum: NtcNr1  Value=NtcNr1.NTCNR_0X0AF  SampleTime=inf
  Enumerated Constant10 : simulink/Sources/Enumerated Constant  RequirementInfo={} %GIDa_b8bf1e8d_a398_47de_9797_4822907a2df7  OutDataTypeStr=Enum: NtcSts1  Value=NtcSts1.NTCSTS_PASSD  SampleTime=inf
  Enumerated Constant13 : simulink/Sources/Enumerated Constant  RequirementInfo={} %GIDa_f80f5832_24ae_4f69_a080_bbb97743b2e1  OutDataTypeStr=Enum: NtcSts1  Value=NtcSts1.NTCSTS_PASSD  SampleTime=inf
  Enumerated Constant14 : simulink/Sources/Enumerated Constant  RequirementInfo={} %GIDa_65c5163a_4e04_4812_814c_26bc4e9ef7e2  OutDataTypeStr=Enum: NtcSts1  Value=NtcSts1.NTCSTS_PASSD  SampleTime=inf
  Enumerated Constant6 : simulink/Sources/Enumerated Constant  RequirementInfo={} %GIDa_d40ee02a_610b_4565_9612_f4584ad3af6d  OutDataTypeStr=Enum: NtcSts1  Value=NtcSts1.NTCSTS_PASSD  SampleTime=inf
  Enumerated Constant7 : simulink/Sources/Enumerated Constant  RequirementInfo={} %GIDa_adb43b73_d23e_4bbf_b22d_731a30ebc358  OutDataTypeStr=Enum: NtcSts1  Value=NtcSts1.NTCSTS_PASSD  SampleTime=inf
  Enumerated Constant9 : simulink/Sources/Enumerated Constant  RequirementInfo={} %GIDa_65085825_93e1_4282_8b88_0f556d313548  OutDataTypeStr=Enum: NtcSts1  Value=NtcSts1.NTCSTS_PASSD  SampleTime=inf
  FutureInput : Constant  RequirementInfo="{'linktype_rmi_doors' '0000bab3 (/E-STEER Core/SubSystem Specifications/Application Functions/SF049A Loss of Assist Manager)' '#SF049A_173' 'true' 'REQ:  SF049A_173' '' } %GIDa_26218168_d286_4969_a9e4_705b653653f0"  Value=false
  NTC_Fault1 : Subsystem  mask(SetNTC){}
      mask help: SetNTC library block
  NTC_Fault2 : Subsystem  mask(SetNTC){}
      mask help: SetNTC library block
  NTC_Fault3 : Subsystem  mask(SetNTC){}
      mask help: SetNTC library block
  NTC_Fault4 : Subsystem  mask(SetNTC){}
      mask help: SetNTC library block
  NTC_Fault5 : Subsystem  mask(SetNTC){}
      mask help: SetNTC library block
  NTC_Fault6 : Subsystem  mask(SetNTC){}
      mask help: SetNTC library block
  SnsrlsMotAgAvl : Outport  RequirementInfo="{'linktype_rmi_doors' '0000bab3 (/E-STEER Core/SubSystem Specifications/Application Functions/SF049A Loss of Assist Manager)' '#SF049A_173' 'true' 'REQ:  SF049A_173' '' } %GIDa_03dc3104_f792_4d3a_8a40_2add4d5ee817"
  wires:
  FutureInput/1 -> SnsrlsMotAgAvl/1  "SnsrlsMotAgAvl"
  Constant17/1 -> Data Store Write5/1
  Constant18/1 -> Data Store Write6/1
  Constant19/1 -> Data Store Write7/1
  Constant20/1 -> Data Store Write8/1
  Enumerated Constant1/1 -> NTC_Fault3/1(NtcNr)
  Constant2/1 -> NTC_Fault3/2(NtcStInfo)
  Enumerated Constant6/1 -> NTC_Fault3/3(NtcSts)
  Constant4/1 -> NTC_Fault3/4(DebStep)
  Enumerated Constant2/1 -> NTC_Fault4/1(NtcNr)
  Constant1/1 -> NTC_Fault4/2(NtcStInfo)
  Enumerated Constant7/1 -> NTC_Fault4/3(NtcSts)
  Constant5/1 -> NTC_Fault4/4(DebStep)
  Enumerated Constant4/1 -> NTC_Fault5/1(NtcNr)
  Constant7/1 -> NTC_Fault5/2(NtcStInfo)
  Enumerated Constant10/1 -> NTC_Fault5/3(NtcSts)
  Constant6/1 -> NTC_Fault5/4(DebStep)
  Enumerated Constant8/1 -> NTC_Fault6/1(NtcNr)
  Constant8/1 -> NTC_Fault6/2(NtcStInfo)
  Enumerated Constant13/1 -> NTC_Fault6/3(NtcSts)
  Constant11/1 -> NTC_Fault6/4(DebStep)
  Enumerated Constant3/1 -> NTC_Fault1/1(NtcNr)
  Constant9/1 -> NTC_Fault1/2(NtcStInfo)
  Enumerated Constant9/1 -> NTC_Fault1/3(NtcSts)
  Constant12/1 -> NTC_Fault1/4(DebStep)
  Constant10/1 -> NTC_Fault2/2(NtcStInfo)
  Enumerated Constant12/1 -> NTC_Fault2/1(NtcNr)
  Enumerated Constant14/1 -> NTC_Fault2/3(NtcSts)
  Constant3/1 -> NTC_Fault2/4(DebStep)

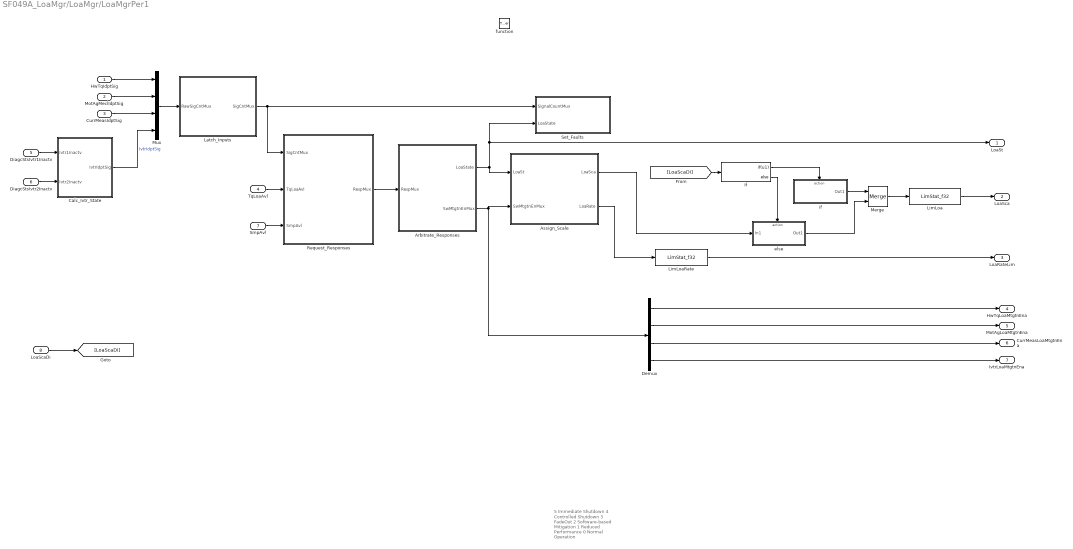
== system SF049A_LoaMgr/LoaMgr/LoaMgrPer1 ==
  note: 5 Immediate Shutdown
      | 4 Controlled Shutdown
      | 3 FadeOut
      | 2 Software-based Mitigation
      | 1 Reduced Performance
      | 0 Normal Operation
  HwTqIdptSig : Inport  RequirementInfo="{'linktype_rmi_doors' '0000bab3 (/E-STEER Core/SubSystem Specifications/Application Functions/SF049A Loss of Assist Manager)' '#SF049A_12' 'true' 'REQ:  SF049A_12' '' } %GIDa_738d9608_1f11_48d9_b5fb_db6b875da4f0"
  MotAgMeclIdptSig : Inport  RequirementInfo="{'linktype_rmi_doors' '0000bab3 (/E-STEER Core/SubSystem Specifications/Application Functions/SF049A Loss of Assist Manager)' '#SF049A_14' 'true' 'REQ:  SF049A_14' '' } %GIDa_2a624495_d7cc_4d20_92e8_f9f8d9f5c9c4"  Port=2
  CurrMeasIdptSig : Inport  RequirementInfo="{'linktype_rmi_doors' '0000bab3 (/E-STEER Core/SubSystem Specifications/Application Functions/SF049A Loss of Assist Manager)' '#SF049A_43' 'true' 'REQ:  SF049A_43' '' } %GIDa_91d29884_2257_4923_b9cb_724eaa988704"  Port=3
  TqLoaAvl : Inport  RequirementInfo={} %GIDa_67da4e6f_783e_4b7f_b2da_bafe95c201fd  Port=4
  DiagcStsIvtr1Inactv : Inport  RequirementInfo="{'linktype_rmi_doors' '0000bab3 (/E-STEER Core/SubSystem Specifications/Application Functions/SF049A Loss of Assist Manager)' '#SF049A_44' 'true' 'REQ:  SF049A_44' '' } %GIDa_d2a02f01_0f9a_4a35_b83d_8146e48af58f"  Port=5
  DiagcStsIvtr2Inactv : Inport  RequirementInfo="{'linktype_rmi_doors' '0000bab3 (/E-STEER Core/SubSystem Specifications/Application Functions/SF049A Loss of Assist Manager)' '#SF049A_184' 'true' 'REQ:  SF049A_184' '' } %GIDa_6476a35b_29d3_4546_be5a_73a3a90db49d"  Port=6
  SmpAvl : Inport  RequirementInfo={} %GIDa_69e486c7_ff85_439f_a16b_5dc177bb9ace  Port=7
  LoaScaDi : Inport  RequirementInfo="{'linktype_rmi_doors' '0000bab3 (/E-STEER Core/SubSystem Specifications/Application Functions/SF049A Loss of Assist Manager)' '#SF049A_202' 'true' 'REQ:  SF049A_202' '' } %GIDa_8444e460_2d30_41ee_8c6a_7225182c7166"  Port=8
  function : TriggerPort  TriggerType=function-call
  Arbitrate_Responses : Subsystem
  Assign_Scale : Subsystem
  Calc_Ivtr_State : Subsystem
  Demux : Demux
  If : If  RequirementInfo="{'linktype_rmi_doors' '0000bab3 (/E-STEER Core/SubSystem Specifications/Application Functions/SF049A Loss of Assist Manager)' '#SF049A_203' 'true' 'REQ:  SF049A_203' '' } %GIDa_c457f394_3d6f_4043_b555_64c59043d4ab"  IfExpression=u1
  Latch_Inputs : Subsystem
  LimLoa : NxtrLim/LimStat_f32  RequirementInfo="{'linktype_rmi_doors' '0000bab3 (/E-STEER Core/SubSystem Specifications/Application Functions/SF049A Loss of Assist Manager)' '#SF049A_110' 'true' 'REQ:  SF049A_110' '' } %GIDa_324c1dd0_d1f9_4e2d_9d54_01262c86ed4e"  LoLim=LOASCAZERO_ULS_F32  HiLim=LOASCAONE_ULS_F32
      settings: AttributesFormatString=|
      | Low Limit: %<LoLim>
      | High Limit:%<HiLim>
  LimLoaRate : NxtrLim/LimStat_f32  RequirementInfo="{'linktype_rmi_doors' '0000bab3 (/E-STEER Core/SubSystem Specifications/Application Functions/SF049A Loss of Assist Manager)' '#SF049A_108' 'true' 'REQ:  SF049A_108' '' } %GIDa_901801f7_af32_4384_938a_193711f98851"  LoLim=LOAMINSLEW_ULSPERSEC_F32  HiLim=LOAMAXSLEW_ULSPERSEC_F32
      settings: AttributesFormatString=|
      | Low Limit: %<LoLim>
      | High Limit:%<HiLim>
  Merge : Merge  RequirementInfo="{'linktype_rmi_doors' '0000bab3 (/E-STEER Core/SubSystem Specifications/Application Functions/SF049A Loss of Assist Manager)' '#SF049A_203' 'true' 'REQ:  SF049A_203' '' } %GIDa_4287e389_3cde_40a6_987d_bc14898a8925"
  Mux : Mux
  Request_Responses : Subsystem
  Set_Faults : Subsystem
  else : Subsystem  RequirementInfo="{'linktype_rmi_doors' '0000bab3 (/E-STEER Core/SubSystem Specifications/Application Functions/SF049A Loss of Assist Manager)' '#SF049A_203' 'true' 'REQ:  SF049A_203' '' } %GIDa_7016a060_e95e_49cf_8bd2_810263e5ad39"  TreatAsAtomicUnit=on
  if : Subsystem  RequirementInfo="{'linktype_rmi_doors' '0000bab3 (/E-STEER Core/SubSystem Specifications/Application Functions/SF049A Loss of Assist Manager)' '#SF049A_203' 'true' 'REQ:  SF049A_203' '' } %GIDa_e6b1d9b0_d725_4b52_92e6_b68ade81a765"  TreatAsAtomicUnit=on
  LoaSt : Outport
  LoaSca : Outport  Port=2
  LoaRateLim : Outport  Port=3
  HwTqLoaMtgtnEna : Outport  RequirementInfo="{'linktype_rmi_doors' '0000bab3 (/E-STEER Core/SubSystem Specifications/Application Functions/SF049A Loss of Assist Manager)' '#SF049A_46' 'true' 'REQ:  SF049A_46' '' } %GIDa_c2717030_0db4_437d_9ad1_5a3a355d0d2d"  Port=4
  MotAgLoaMtgtnEna : Outport  RequirementInfo="{'linktype_rmi_doors' '0000bab3 (/E-STEER Core/SubSystem Specifications/Application Functions/SF049A Loss of Assist Manager)' '#SF049A_47' 'true' 'REQ:  SF049A_47' '' } %GIDa_26ce4f86_4a2a_41f4_9309_52885d709c62"  Port=5
  CurrMeasLoaMtgtnEna : Outport  RequirementInfo="{'linktype_rmi_doors' '0000bab3 (/E-STEER Core/SubSystem Specifications/Application Functions/SF049A Loss of Assist Manager)' '#SF049A_48' 'true' 'REQ:  SF049A_48' '' } %GIDa_1fd35a83_f605_4b7d_98e6_d5eadefd8386"  Port=6
  IvtrLoaMtgtnEna : Outport  RequirementInfo="{'linktype_rmi_doors' '0000bab3 (/E-STEER Core/SubSystem Specifications/Application Functions/SF049A Loss of Assist Manager)' '#SF049A_49' 'true' 'REQ:  SF049A_49' '' } %GIDa_103e57d6_8a6f_4228_b378_4c12f8abfa9c"  Port=7
  wires:
  HwTqIdptSig/1 -> Mux/1
  Mux/1 -> Latch_Inputs/1(RawSigCntMux)
  Calc_Ivtr_State/1(IvtrIdptSig) -> Mux/4  "IvtrIdptSig"
  CurrMeasIdptSig/1 -> Mux/3
  DiagcStsIvtr1Inactv/1 -> Calc_Ivtr_State/1(Ivtr1Inactv)
  DiagcStsIvtr2Inactv/1 -> Calc_Ivtr_State/2(Ivtr2Inactv)
  MotAgMeclIdptSig/1 -> Mux/2
  Latch_Inputs/1(SigCntMux) -> Set_Faults/1(SignalCountMux), Request_Responses/1(SigCntMux)
  TqLoaAvl/1 -> Request_Responses/2(TqLoaAvl)
  SmpAvl/1 -> Request_Responses/3(SmpAvl)
  Request_Responses/1(RespMux) -> Arbitrate_Responses/1(RespMux)
  Arbitrate_Responses/1(LoaState) -> Set_Faults/2(LoaState), LoaSt/1, Assign_Scale/1(LoaSt)
  Arbitrate_Responses/2(SwMtgtnEnMux) -> Demux/1, Assign_Scale/2(SwMtgtnEnMux)
  Demux/1 -> HwTqLoaMtgtnEna/1
  Demux/3 -> CurrMeasLoaMtgtnEna/1
  Demux/2 -> MotAgLoaMtgtnEna/1
  Demux/4 -> IvtrLoaMtgtnEna/1
  Assign_Scale/2(LoaRate) -> LimLoaRate/1
  LimLoaRate/1 -> LoaRateLim/1
  LoaScaDi/1 -> [LoaScaDi]
  LimLoa/1 -> LoaSca/1
  If/1 -> if/Action
  If/2 -> else/Action
  if/1(Out1) -> Merge/1
  else/1(Out1) -> Merge/2
  Merge/1 -> LimLoa/1
  Assign_Scale/1(LoaSca) -> else/1(In1)
  [LoaScaDi] -> If/1

== system SF049A_LoaMgr/ISO Fault Debounce/DiagMgr/CopyRight2 ==

== system SF049A_LoaMgr/ISO Fault Debounce/DiagMgr/If Action Subsystem ==
  EA : Inport
  Qlf : Inport  Port=2
  Action Port : ActionPort  ActionType=else
  EAo : Outport
  Qlfo : Outport  Port=2
  wires:
  EA/1 -> EAo/1
  Qlf/1 -> Qlfo/1

== system SF049A_LoaMgr/ISO Fault Debounce/DiagMgr/If Action Subsystem1 ==
  Qlf : Inport
  EA : Inport  Port=2
  Action Port : ActionPort  ActionType=then
  Qlfo : Outport
  EAo : Outport  Port=2
  wires:
  EA/1 -> EAo/1
  Qlf/1 -> Qlfo/1

== system SF049A_LoaMgr/ISO Fault Debounce/DiagMgr/If Action Subsystem3 ==
  In1 : Inport
  Action Port : ActionPort  ActionType=then
  Out1 : Outport
  wires:
  In1/1 -> Out1/1

== system SF049A_LoaMgr/ISO Fault Debounce/DiagMgr/If Action Subsystem4 ==
  In1 : Inport
  Action Port : ActionPort  ActionType=else
  Out1 : Outport
  wires:
  In1/1 -> Out1/1

== system SF049A_LoaMgr/ISO Fault Debounce/DiagMgr/NTCSTS_FAILD ==
  EA : Inport
  Qlf : Inport  Port=2
  Action Port : ActionPort  ActionType=case
  EAo : Outport
  Qlfo : Outport  Port=2
  wires:
  EA/1 -> EAo/1
  Qlf/1 -> Qlfo/1

== system SF049A_LoaMgr/ISO Fault Debounce/DiagMgr/NTCSTS_PASSD ==
  EA : Inport
  Qlf : Inport  Port=2
  Action Port : ActionPort  ActionType=case
  EAo : Outport
  Qlfo : Outport  Port=2
  wires:
  EA/1 -> EAo/1
  Qlf/1 -> Qlfo/1

== system SF049A_LoaMgr/ISO Fault Debounce/DiagMgr/NTCSTS_PREFAILD ==
  EA : Inport
  DS : Inport  Port=2
  TS : Inport  Port=3
  Qlf : Inport  Port=4
  Action Port : ActionPort  ActionType=case
  CopyRight2 : Subsystem  Description=|  mask(Copyright Information){none=on}
      | Copyright info block.                                               
      |                                                                     
      | Place copyright information at the top of every subsystem in design.
      mask prompts: none "No parameters"
      mask help: Place copyright information at the top of every subsystem in design.
      mask Display:
      | NxtrConf = 'Nexteer Confidential';
      | 
      | sys = bdroot; %handle for the current model ("system")
      | first = get_param(sys,'Created');
      | first = first(end-3:end);  %year is last four digits
      | 
      | last = get_param(sys,'LastModifiedDate');
      | if isempty(last)
      |     last = datestr(now,'yyyy');
      | else
      |     last = last(end-3:end);
      | end
      | 
      | if strcmp(first,last)
      |     fprintf('%s -- Copyright %s Nexteer',NxtrConf,first)
      | else
      |     fprintf('%s -- %s%s- %s Nexteer',NxtrConf,char(169),first,last)
      | end
  Data Type Conversion : DataTypeConversion
  If : If  IfExpression=u1 <= 0
  If Action Subsystem : Subsystem  TreatAsAtomicUnit=on
  If Action Subsystem1 : Subsystem  TreatAsAtomicUnit=on
  Merge : Merge
  Merge1 : Merge
  EAo : Outport
  Qlfo : Outport  Port=2
  wires:
  EA/1 -> If Action Subsystem1/2(EA), If/1
  If/1 -> If Action Subsystem/Action
  If/2 -> If Action Subsystem1/Action
  DS/1 -> Data Type Conversion/1, If Action Subsystem1/1(DS)
  TS/1 -> If Action Subsystem1/4(TS)
  If Action Subsystem/1(EAo) -> Merge/1
  If Action Subsystem1/1(EAo) -> Merge/2
  If Action Subsystem1/2(Qlfo) -> Merge1/2
  If Action Subsystem/2(Qlfo) -> Merge1/1
  Merge/1 -> EAo/1
  Merge1/1 -> Qlfo/1
  Qlf/1 -> If Action Subsystem/2(Qlf), If Action Subsystem1/3(Qlf)
  Data Type Conversion/1 -> If Action Subsystem/1(DS)
